simulink model "LUPAhoming"  (R2024a)
settings: Solver=FixedStepAuto  StartTime=0.0  StopTime=inf  FixedStep=0.001  RelTol=1e-3
values from neighbouring files (symbols this model uses):
  C = 258.803991051052    (= 258.803991051)    [Constants_3Body_v2.m]
libraries: slrealtimeethercatlib x7
settings Model: Creator=Bosma  LastModifiedBy=Bosma
settings SolverCC: ConcurrentTasks=on  PositivePriorityOrder=on
settings OptimizationCC: BlockReduction=off  OptimizeBlockIOStorage=off
settings DebuggingCC: TasksWithSamePriorityMsg=none
settings HardwareCC: ProdBitPerLong=64  ProdLongLongMode=on  ProdHWDeviceType=Intel->x86-64 (Linux 64)
settings RTWCC: Description=Speedgoat Real-Time Target Machine  SystemTargetFile=speedgoat.tlc  TemplateMakefile=slrealtime_default_tmf  Toolchain=Simulink Real-Time Toolchain  BuildConfiguration=Faster Runs  CodeExecutionProfiling=on  TargetLang=C++
settings SimulinkRealTimeTargetCC: InstructionSetFMA=off  LogToMDFFile=off

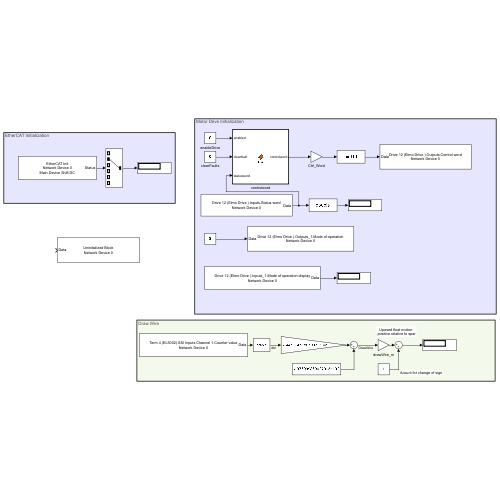
[thumbnail: Simulink's stored preview of the top-level diagram]
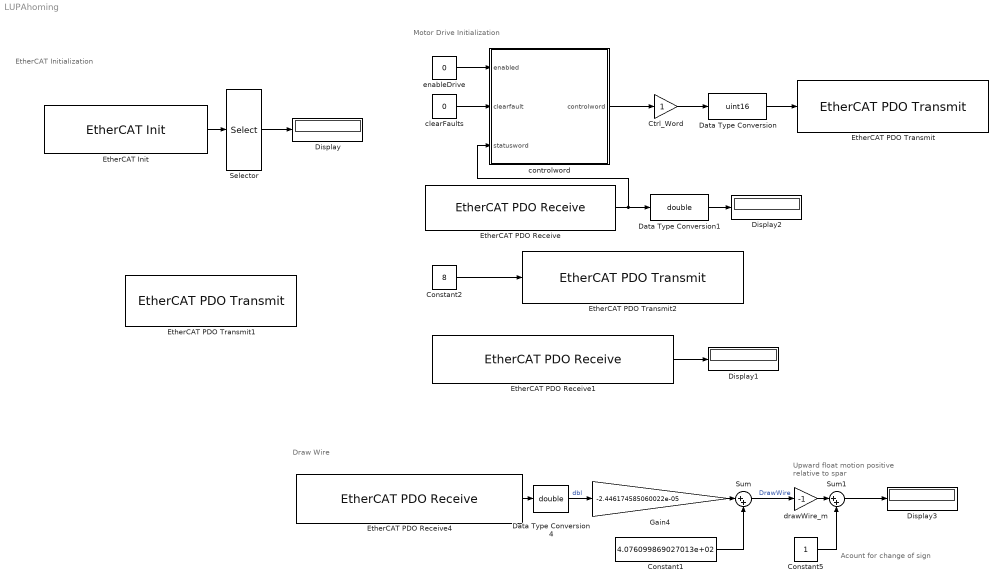
== system LUPAhoming ==
  note: EtherCAT Initialization
  note: Motor Drive Initialization
  note: Draw Wire
  note: Acount for change of sign
  note: Upward float motion
      | positive relative to spar
  Constant1 : Constant  Value=4.076099869027013e+02
  Constant2 : Constant  Value=8  OutDataTypeStr=int8
  Constant5 : Constant
  Ctrl_Word : Gain
  Data Type Conversion : DataTypeConversion  OutDataTypeStr=uint16  SaturateOnIntegerOverflow=off  RndMeth=Floor
  Data Type Conversion1 : DataTypeConversion  OutDataTypeStr=double  SaturateOnIntegerOverflow=off  RndMeth=Floor
  Data Type Conversion4 : DataTypeConversion  OutDataTypeStr=double  SaturateOnIntegerOverflow=off  RndMeth=Floor
  Display{,1..3} (4 alike) : Display
  EtherCAT Init : slrealtimeethercatlib/EtherCAT Init  Priority=0  config_file=C:\2024\Software\LUPA\Simulink\EtherCAT\LUPA1kHz.xml  device_id=0  portnum=1  initstate=2  dctuning=0  enaDebug=0  logFile='c:\dbglog.txt'  sample_time=0.001000  DCMode=2
  EtherCAT PDO Receive : slrealtimeethercatlib/EtherCAT PDO Receive  Priority=2  sig_name=Drive 12 (Elmo Drive ).Inputs.Status word  sig_offset=1824  sig_type=uint16  type_size=16  sig_dim=1  device_id=0  sample_time=0.001000
  EtherCAT PDO Receive1 : slrealtimeethercatlib/EtherCAT PDO Receive  Priority=2  sig_name=Drive 12 (Elmo Drive ).Inputs_1.Mode of operation display  sig_offset=1840  sig_type=int8  type_size=8  sig_dim=1  device_id=0  sample_time=0.001000
  EtherCAT PDO Receive4 : slrealtimeethercatlib/EtherCAT PDO Receive  Priority=2  sig_name=Term 4 (EL5002).SSI Inputs Channel 1.Counter value  sig_offset=1384  sig_type=uint32  type_size=32  sig_dim=1  device_id=0  sample_time=0.001000
  EtherCAT PDO Transmit : slrealtimeethercatlib/EtherCAT PDO Transmit  Priority=3  sig_name=Drive 12 (Elmo Drive ).Outputs.Control word  sig_offset=1824  sig_type=uint16  type_size=16  sig_dim=1  device_id=0  sample_time=0.001000
  EtherCAT PDO Transmit1 : slrealtimeethercatlib/EtherCAT PDO Transmit  Priority=3  sig_offset=1  sig_type=boolean  type_size=1  sig_dim=1  device_id=0  sample_time=1
  EtherCAT PDO Transmit2 : slrealtimeethercatlib/EtherCAT PDO Transmit  Priority=3  sig_name=Drive 12 (Elmo Drive ).Outputs_1.Mode of operation  sig_offset=1840  sig_type=int8  type_size=8  sig_dim=1  device_id=0  sample_time=0.001000
  Gain4 : Gain  Gain=-2.446174585060022e-05
  Selector : Selector  InputPortWidth=6  IndexOptions=Index vector (dialog)  Indices=[2]  OutputSizes=1
  Sum : Sum  Inputs=|++
  Sum1 : Sum  Inputs=|++
  clearFaults : Constant  Value=0
  controlword : MATLAB Function  TreatAsAtomicUnit=on
  drawWire_m : Gain  Gain=-1
  enableDrive : Constant  Value=0
  wires:
  EtherCAT Init/1 -> Selector/1
  Selector/1 -> Display/1
  enableDrive/1 -> controlword/1(enabled)
  Data Type Conversion1/1 -> Display2/1
  Data Type Conversion/1 -> EtherCAT PDO Transmit/1
  Ctrl_Word/1 -> Data Type Conversion/1
  EtherCAT PDO Receive/1 -> Data Type Conversion1/1, controlword/3(statusword)
  controlword/1(controlword) -> Ctrl_Word/1
  EtherCAT PDO Receive1/1 -> Display1/1
  clearFaults/1 -> controlword/2(clearfault)
  Constant2/1 -> EtherCAT PDO Transmit2/1
  drawWire_m/1 -> Sum1/1
  Constant5/1 -> Sum1/2
  EtherCAT PDO Receive4/1 -> Data Type Conversion4/1
  Data Type Conversion4/1 -> Gain4/1  "dbl"
  Constant1/1 -> Sum/2
  Sum1/1 -> Display3/1
  Gain4/1 -> Sum/1
  Sum/1 -> drawWire_m/1  "DrawWire"

== matlab function LUPAhoming/controlword ==
  data: enabled input; clearfault input; statusword input; controlword output
function controlword = fcn(enabled, clearfault, statusword)

bitstatus = bitget(statusword,1:16);

if ~clearfault
    if enabled
        if bitstatus(1) == 0 % Ready to switch on not ready
            controlword = 6; % command ready switch on
        elseif ~bitstatus(2) % switched not yet on
            controlword = 7; % command switch on
        elseif ~bitstatus(3) % operation not yet enabled
            controlword = 15; % command enable
        else
            controlword = 15; % maintain enabled state
        end
    else
        controlword = 4; % command disabled
    end
else
    controlword = 128; % command clear faults
end
